simulink model "plant_test"  (R2023b)
settings: Solver=VariableStepAuto  StartTime=0.0  StopTime=t_end  RelTol=1e-3
values from neighbouring files (symbols this model uses):
  dt = (2*pi)/(100*w)    [plot_bode.m]    (also in plot_impulse.m = 0.001; plot_initial.m = 0.001)
  param = plant_param()    [plot_bode.m]    (also in plot_impulse.m; plot_initial.m)
  sysc = plant_sysc(param)    [plot_bode.m]    (also in plot_impulse.m; plot_initial.m)
  w = w_vec(i)    [plot_bode.m]
  x0 = [0;0]    [plot_bode.m]    (also in plot_impulse.m; plot_initial.m = [1;0])
undefined symbols (not defined in the file or in its folder): ue, xe
libraries: fl_lib x7, nesl_utility x4
settings Model: Creator=MPC5  LastModifiedBy=MPC5

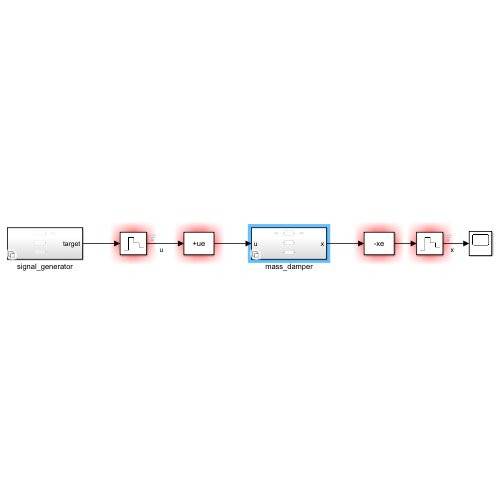
[thumbnail: Simulink's stored preview of the top-level diagram]
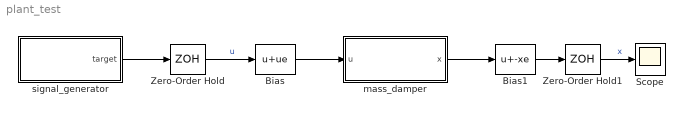
== system plant_test ==
  Bias : Bias  Bias=ue  SaturateOnIntegerOverflow=off
  Bias1 : Bias  Bias=-xe  SaturateOnIntegerOverflow=off
  Scope : Scope
  Zero-Order Hold : ZeroOrderHold  SampleTime=dt
  Zero-Order Hold1 : ZeroOrderHold  SampleTime=dt
  mass_damper : Subsystem  Variant=on
  signal_generator : Subsystem  Variant=on
  wires:
  Zero-Order Hold/1 -> Bias/1  "u"
  Bias/1 -> mass_damper/1(u)
  mass_damper/1(x) -> Bias1/1
  Zero-Order Hold1/1 -> Scope/1  "x"
  signal_generator/1(target) -> Zero-Order Hold/1
  Bias1/1 -> Zero-Order Hold1/1

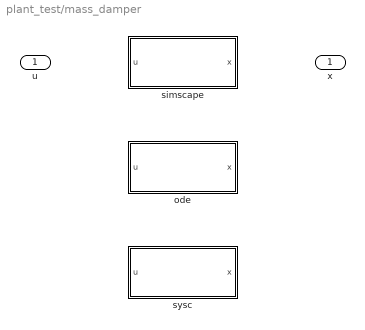
== system plant_test/mass_damper ==
  u : Inport
  ode : Subsystem  VariantControl="plant_model_type==\"ode\""
  simscape : Subsystem  VariantControl="plant_model_type==\"simscape\""
  sysc : Subsystem  VariantControl="plant_model_type==\"sysc\""
  x : Outport

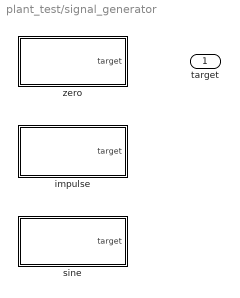
== system plant_test/signal_generator ==
  impulse : Subsystem  VariantControl="input_signal_type==\"impulse\""
  sine : Subsystem  VariantControl="input_signal_type==\"sine\""
  zero : Subsystem  VariantControl="input_signal_type==\"zero\""
  target : Outport

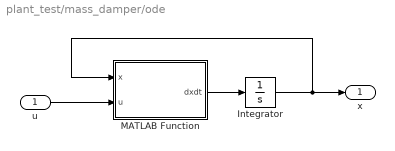
== system plant_test/mass_damper/ode ==
  u : Inport
  Integrator : Integrator  InitialCondition=x0
  MATLAB Function : MATLAB Function  TreatAsAtomicUnit=on
  x : Outport
  wires:
  MATLAB Function/1(dxdt) -> Integrator/1
  u/1 -> MATLAB Function/2(u)
  Integrator/1 -> x/1, MATLAB Function/1(x)

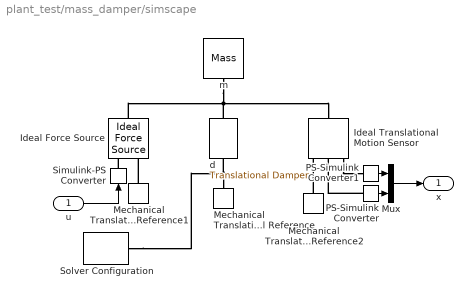
== system plant_test/mass_damper/simscape ==
  u : Inport
  Ideal Force Source : fl_lib/Mechanical/Mechanical Sources/Ideal Force Source
  Ideal Translational Motion Sensor : fl_lib/Mechanical/Mechanical Sensors/Ideal Translational Motion Sensor  reference=foundation.enum.MeasurementReference.difference  acceleration_port=false  velocity_port=true  position_port=true  offset=x0(1) m
  Mechanical Translational Reference : fl_lib/Mechanical/Translational Elements/Mechanical Translational Reference
  Mechanical Translational Reference1 : fl_lib/Mechanical/Translational Elements/Mechanical Translational Reference
  Mechanical Translational Reference2 : fl_lib/Mechanical/Translational Elements/Mechanical Translational Reference
  Mux : Mux  Inputs=2
  PS-Simulink Converter : nesl_utility/PS-Simulink Converter  PhysicalDomain=network_engine_domain  SubClassName=ps_output  LeftPortType=input  RightPortType=output  PseudoPeriodic=off  Frequencies=[]  VectorFormat=inherit  Unit=inherit  AffineConversion=off
  PS-Simulink Converter1 : nesl_utility/PS-Simulink Converter  PhysicalDomain=network_engine_domain  SubClassName=ps_output  LeftPortType=input  RightPortType=output  PseudoPeriodic=off  Frequencies=[]  VectorFormat=inherit  Unit=inherit  AffineConversion=off
  Simulink-PS Converter : nesl_utility/Simulink-PS Converter  PhysicalDomain=network_engine_domain  SubClassName=ps_input  LeftPortType=input  RightPortType=output  PseudoPeriodic=off  Frequencies=[]  NoiseDistribution=none  NoiseParameters=[]  Unit=1  AffineConversion=off  FilteringAndDerivatives=provide  SimscapeFilterOrder=1  InputFilterTimeConstant=0.001  UdotUserProvided=0
  Solver Configuration : nesl_utility/Solver Configuration  PhysicalDomain=network_engine_domain  SubClassName=solver  LeftPortType=input  RightPortType=generic  Tones=[]  Harmonics=[]  SimulateNoise=off  Profile=off  UseLocalSampling=off  EnableSwitchedLinearOptims=on  FrequencyDomain=off  UseCCode=off  RelTol=0.001  AbsTol=0.001  MinStep=1e-09  ToWorkspace=off  RevertToSquareIcSolve=off  NumHomotopyIterations=100  PhasorMode=off  PhasorModeNumHarmonics=1  ConsistencySolver=NEWTON_XTOL_AFTER_FTOL  IndexReductionMethod=DerivativeReplacement  DoDC=off  ResidualTolerance=1e-09  ConsistencyTolSource=GLOBAL  ConsistencyAbsTol=0.001  ConsistencyRelTol=0.001  ConsistencyTolFactor=0.001  UseLocalSolver=off  LocalSolverChoice=NE_BACKWARD_EULER_ADVANCER  ResolveIndetEquations=on  FunctionEvalNumThread=1  LocalSolverSampleTime=0.001  DoFixedCost=off  MaxNonlinIter=3  MaxModeIter=2  ComputeImpulses=off  ImpulseIterations=2  LinearAlgebra=auto  LinearAlgebraNumThread=0  EquationFormulation=NE_TIME_EF  DelaysMemoryBudget=1024  AutomaticFiltering=on  FilteringTimeConstant=0.001  PartitionStorageMethod=AS_NEEDED  PartitionMemoryBudget=1024  PartitionMethod=ROBUST  MultibodyUseLocalSolver=off  MultibodyLocalSolverChoice=ODE1  MultibodyLocalSolverSampleTime=0.001
  d : fl_lib/Mechanical/Translational Elements/Translational Damper  D=param.d N*s/m  v_specify=off  v_priority=High  v=x0(2) m/s  v_nominal_specify=off  v_nominal_unit=m/s  v_nominal_value=1  f_specify=off  f_priority=None  f=0 N  f_nominal_specify=off  f_nominal_unit=N  f_nominal_value=1
  m : fl_lib/Mechanical/Translational Elements/Mass  mass=param.m kg  num_ports=foundation.enum.numPorts2.one  v_specify=on  v_priority=High  v=x0(2) m/s  v_nominal_specify=off  v_nominal_unit=m/s  v_nominal_value=1  f_specify=off  f_priority=None  f=0 N  f_nominal_specify=off  f_nominal_unit=N  f_nominal_value=1
  x : Outport
  wires:
  Mux/1 -> x/1
  PS-Simulink Converter1/1 -> Mux/1
  u/1 -> Simulink-PS Converter/1
  PS-Simulink Converter/1 -> Mux/2
  connections:
  m/LConn1 -- d/LConn1 -- Ideal Force Source/LConn1 -- Ideal Translational Motion Sensor/LConn1
  d/RConn1 -- Mechanical Translational Reference/LConn1 -- Solver Configuration/RConn1
  Ideal Translational Motion Sensor/RConn3 -- PS-Simulink Converter1/LConn1
  Mechanical Translational Reference1/LConn1 -- Ideal Force Source/RConn2
  Mechanical Translational Reference2/LConn1 -- Ideal Translational Motion Sensor/RConn1
  PS-Simulink Converter/LConn1 -- Ideal Translational Motion Sensor/RConn2
  Simulink-PS Converter/RConn1 -- Ideal Force Source/RConn1

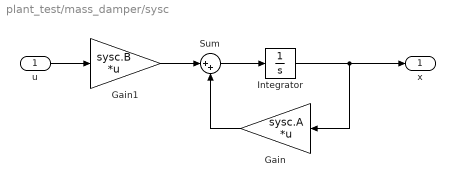
== system plant_test/mass_damper/sysc ==
  u : Inport
  Gain : Gain  Gain=sysc.A  Multiplication=Matrix(K*u)
  Gain1 : Gain  Gain=sysc.B  Multiplication=Matrix(K*u)
  Integrator : Integrator  InitialCondition=x0
  Sum : Sum  Inputs=|++
  x : Outport
  wires:
  Sum/1 -> Integrator/1
  u/1 -> Gain1/1
  Gain1/1 -> Sum/1
  Gain/1 -> Sum/2
  Integrator/1 -> x/1, Gain/1

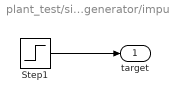
== system plant_test/signal_generator/impulse ==
  Step1 : Step  Time=1e-2  Before=100  After=0  SampleTime=0
  target : Outport
  wires:
  Step1/1 -> target/1

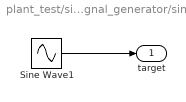
== system plant_test/signal_generator/sine ==
  Sine Wave1 : Sin  Amplitude=0.1  Frequency=w  SampleTime=0
  target : Outport
  wires:
  Sine Wave1/1 -> target/1

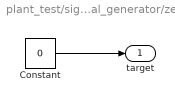
== system plant_test/signal_generator/zero ==
  Constant : Constant  Value=0
  target : Outport
  wires:
  Constant/1 -> target/1

== matlab function plant_test/mass_damper/ode/MATLAB Function ==
  data: x input size=param.xdim; u input size=param.udim; dxdt output size=param.xdim; param parameter
function dxdt = ode(x,u,param)
    dxdt = plant_ode(0,x,u,param);
end
